simulink subsystem "fifo"  (R2023a)
settings: Solver=VariableStepAuto  StartTime=0.0  StopTime=10.0  RelTol=1e-3
libraries: hdlsllib x1
settings Model: Creator=harry  LastModifiedBy=harry

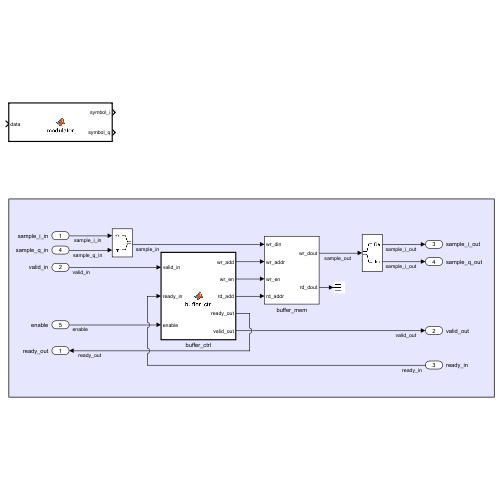
[thumbnail: Simulink's stored preview of the top-level diagram]
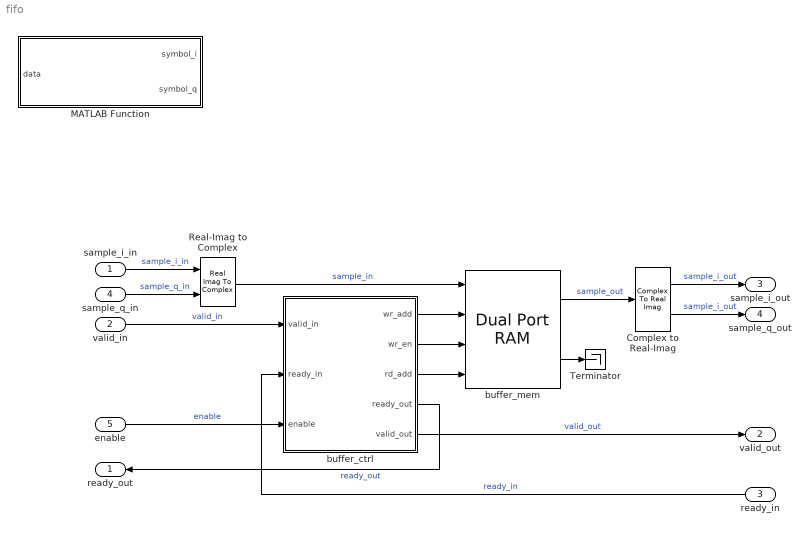
== system fifo ==
  sample_i_in : Inport  OutDataTypeStr=fixdt(1,16,15)
  valid_in : Inport  Port=2  OutDataTypeStr=boolean
  ready_in : Inport  Port=3  OutDataTypeStr=boolean
  sample_q_in : Inport  Port=4  OutDataTypeStr=fixdt(1,16,15)
  enable : Inport  Port=5  OutDataTypeStr=boolean
  Complex to Real-Imag : ComplexToRealImag
  MATLAB Function : MATLAB Function
      settings: MinAlgLoopOccurrences=on
  Real-Imag to Complex : RealImagToComplex
  Terminator : Terminator
  buffer_ctrl : MATLAB Function  TreatAsAtomicUnit=on
  buffer_mem : hdlsllib/HDL RAMs/Dual Port RAM  ram_size=10
  ready_out : Outport  OutDataTypeStr=boolean
  valid_out : Outport  Port=2  OutDataTypeStr=boolean
  sample_i_out : Outport  Port=3  OutDataTypeStr=fixdt(1,16,15)
  sample_q_out : Outport  Port=4  OutDataTypeStr=fixdt(1,16,15)
  wires:
  buffer_ctrl/1(wr_add) -> buffer_mem/2
  buffer_ctrl/2(wr_en) -> buffer_mem/3
  buffer_ctrl/3(rd_add) -> buffer_mem/4
  sample_i_in/1 -> Real-Imag to Complex/1  "sample_i_in"
  buffer_ctrl/4(ready_out) -> ready_out/1  "ready_out"
  valid_in/1 -> buffer_ctrl/1(valid_in)  "valid_in"
  ready_in/1 -> buffer_ctrl/2(ready_in)  "ready_in"
  buffer_ctrl/5(valid_out) -> valid_out/1  "valid_out"
  sample_q_in/1 -> Real-Imag to Complex/2  "sample_q_in"
  Real-Imag to Complex/1 -> buffer_mem/1  "sample_in"
  buffer_mem/1 -> Complex to Real-Imag/1  "sample_out"
  Complex to Real-Imag/1 -> sample_i_out/1  "sample_i_out"
  Complex to Real-Imag/2 -> sample_q_out/1  "sample_i_out"
  buffer_mem/2 -> Terminator/1
  enable/1 -> buffer_ctrl/3(enable)  "enable"

== matlab function fifo/buffer_ctrl ==
  data: valid_in input; wr_add output; wr_en output; rd_add output; ready_in input; ready_out output; valid_out output; enable input
function [wr_add, wr_en, rd_add, ready_out, valid_out] = buffer_ctrl(valid_in, ready_in, enable)

    %----------------------------------------------------------------------
    % TYPES DEFINITION
    %----------------------------------------------------------------------
    std_10 = numerictype(0,10,0);

    %----------------------------------------------------------------------
    % REGISTERS DEFINITION
    %----------------------------------------------------------------------
    persistent wr_add_reg;
    if isempty(wr_add_reg)
        wr_add_reg = fi(0, std_10);  % Must initialize with fixed size/type
    end

    persistent rd_add_reg;
    if isempty(rd_add_reg)
        rd_add_reg = fi(0, std_10);  % Must initialize with fixed size/type
    end

    persistent cnt_reg;
    if isempty(cnt_reg)
        cnt_reg = fi(0, std_10);  % Must initialize with fixed size/type
    end
    %----------------------------------------------------------------------
    % ASSIGNATION DEFINITION
    %----------------------------------------------------------------------
    wr_add = wr_add_reg;
    rd_add = rd_add_reg;
    cnt    = cnt_reg;
    wr_en  = valid_in && enable;

    %----------------------------------------------------------------------
    % PROCESS DEFINITION
    %----------------------------------------------------------------------
    % Write pointer
    if (enable)
        if (valid_in)
            if (wr_add_reg == fi(1023, std_10))
                wr_add_reg = fi(0, std_10);
            else
                inc = wr_add_reg + 1;
                wr_add_reg = fi(inc, std_10);
            end
        end
    else
        wr_add_reg = fi(0, std_10);
    end

    % Read pointer
    if (enable)
        if (ready_in)
            if (rd_add_reg == fi(1023, std_10))
                rd_add_reg = fi(0, std_10);
            else
                inc = rd_add_reg + 1;
                rd_add_reg = fi(inc, std_10);
            end
        end
    else
        rd_add_reg = fi(0, std_10);
    end

    % Data number counter in Fifo
    if (enable)
        if (ready_in && not(valid_in))
            dec = cnt_reg - 1;
            cnt_reg = fi(dec, std_10);
        elseif (not(ready_in) && valid_in)
            inc = cnt_reg + 1;
            cnt_reg = fi(inc, std_10);
        end
    else
        cnt_reg = fi(0, std_10);
    end

    % generate ready_out
    if (enable)
        if (cnt > fi(1000, std_10))
            ready_out = false;
        else
            ready_out = true;
        end
    else
        ready_out = false;
    end

    % generate valid_out
    if (enable)
        if (cnt > fi(0, std_10))
            valid_out = true;
        else
            valid_out = false;
        end
    else
        valid_out = false;
    end

end

== matlab function fifo/MATLAB Function ==
  data: data input; symbol_i output; symbol_q output
function [symbol_i, symbol_q] = modulator(data)

    %----------------------------------------------------------------------
    % TYPES DEFINITION
    %----------------------------------------------------------------------
    sig_16_15 = numerictype(1,16,15);
    c_sqrt2dv2 = fi((sqrt(2)/2), sig_16_15);

    %----------------------------------------------------------------------
    % REGISTERS DEFINITION
    %----------------------------------------------------------------------
    
    %----------------------------------------------------------------------
    % ASSIGNATION DEFINITION
    %----------------------------------------------------------------------
    switch data
        case fi(0, 0, 2, 0)
            symbol_i = +c_sqrt2dv2;
            symbol_q = +c_sqrt2dv2;
        case fi(1, 0, 2, 0)
            symbol_i = -c_sqrt2dv2;
            symbol_q = +c_sqrt2dv2;
        case fi(2, 0, 2, 0)
            symbol_i = -c_sqrt2dv2;
            symbol_q = -c_sqrt2dv2;
        case fi(2, 0, 2, 0)
            symbol_i = +c_sqrt2dv2;
            symbol_q = -c_sqc_sqrt2dv2rt2;        
    end

    %----------------------------------------------------------------------
    % PROCESS DEFINITION
    %----------------------------------------------------------------------
end
